simulink model "Final_Microgrid_Ssstem"  (R2021a)
settings: Solver=VariableStepAuto  StartTime=0.0  StopTime=.2  RelTol=1e-3
undefined symbols (not defined in the file): Acid, Lead
libraries: spsIGBTDiodeLib x6, spsSeriesRLCBranchLib x3, spsVoltageMeasurementLib x3, spsCurrentMeasurementLib x2, spsACVoltageSourceLib x1, spsBatteryLib x1, pid_lib x1, spsPLLLib x1, spsPWMGeneratorDCDCLib x1, spspowerguiLib x1
settings Model: Creator=User  LastModifiedBy=User
settings SolverCC: AlgebraicLoopSolver=TrustRegion
settings DataIOCC: ReturnWorkspaceOutputs=off
settings DebuggingCC: SFMachineParentedDataDiag=warning  ArithmeticOperatorsInVariantConditions=warning
settings SFSimCC: SimUseLocalCustomCode=off  CustomCodeUndefinedFunction=UseInterfaceOnly
settings RTWCC: RTWUseLocalCustomCode=off

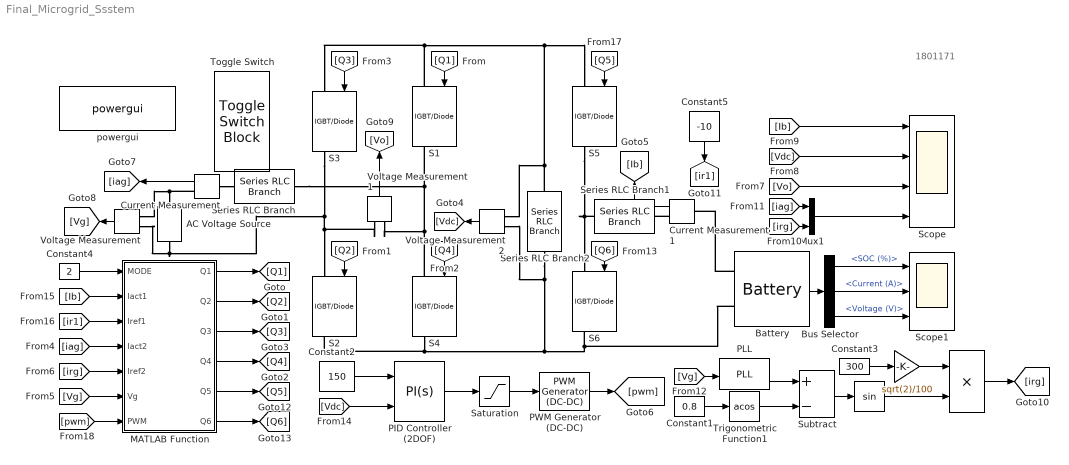
== system Final_Microgrid_Ssstem ==
  note: 1801171
  " " : Product
  "  " : Gain  Gain=sqrt(2)/100
  "   " : Trigonometry
  AC Voltage Source : spsACVoltageSourceLib/AC Voltage Source  Amplitude=100*sqrt(2)  Phase=0  Frequency=50  SampleTime=0  Measurements=None  BusType=swing  Pref=10e3  Qref=0  Qmin=-inf  Qmax=+inf
  Battery : spsBatteryLib/Battery  BatType=Lead-Acid  ShowTempParam=off  ThermalPreset=no  ShowAgeParam=off  NomV=60  NomQ=5.4  SOC=100  Batt_Tr=30  PresetModel=off  MaxQ=5.4  MinV=45  FullV=80  Dis_rate=2.3478  R=0.013333  Normal_OP=4.8835  expZone="[70      0.2653]"  current=[6.5 13 32.5]  Units=Time  Tci=20  NomT=20  T2=-30  MaxQ2=4.8  FullV2=7.1  Normal_OP2=5.655  expZone2="[6.58           1]"  Rca=0.6  ti=2000  Dp=0  Neq0=0  Tsim=1e6  Ta1=25  Qeol=5.4*0.9  Reol=0.013333*1.2  Char_age=[2.3478, 3]  Dis_age=[2.3478, 10]  N1=1500  N2=10500  N3=1000  N4=1400  Ta2=45  N5=950
  Bus Selector : BusSelector  OutputSignals=SOC (%),Current (A),Voltage (V)
  Constant1 : Constant  Value=0.8
  Constant2 : Constant  Value=150
  Constant3 : Constant  Value=300
  Constant4 : Constant  Value=2
  Constant5 : Constant  Value=-10
  Current Measurement : spsCurrentMeasurementLib/Current Measurement  PhasorSimulation=off  OutputType=Complex  PSBequivalent=0
  Current Measurement1 : spsCurrentMeasurementLib/Current Measurement  PhasorSimulation=off  OutputType=Complex  PSBequivalent=0
  MATLAB Function : MATLAB Function  TreatAsAtomicUnit=on
  Mux1 : Mux  Inputs=2
  PID Controller (2DOF) : pid_lib/PID Controller (2DOF)  Controller=PI  Form=Parallel  TimeDomain=Continuous-time  UseExternalTs=off  SampleTime=-1  IntegratorMethod=Forward Euler  FilterMethod=Forward Euler  ControllerParametersSource=internal  P=0.1  I=0.01  D=0  UseFilter=on  N=100  b=1  c=1  TunerSelectOption=Transfer Function Based (PID Tuner App)  InitialConditionSource=internal  InitialConditionForIntegrator=0  InitialConditionForFilter=0  DifferentiatorICPrevScaledInput=0  ExternalReset=none  TrackingMode=off  Kt=1  LimitOutput=off  SatLimitsSource=internal  UpperSaturationLimit=inf  LowerSaturationLimit=-inf  LinearizeAsGain=on  AntiWindupMode=none  Kb=1  POutMin=[]  POutMax=[]  IOutMin=[]  IOutMax=[]  DOutMin=[]  DOutMax=[]  NOutMin=[]  NOutMax=[]  bOutMin=[]  bOutMax=[]  cOutMin=[]  cOutMax=[]  SumOutMin=[]  SumOutMax=[]  SaturationOutMin=[]  SaturationOutMax=[]  PParamMin=[]  PParamMax=[]  IParamMin=[]  IParamMax=[]  DParamMin=[]  DParamMax=[]  NParamMin=[]  NParamMax=[]  bParamMin=[]  bParamMax=[]  cParamMin=[]  cParamMax=[]  KbParamMin=[]  KbParamMax=[]  KtParamMin=[]  KtParamMax=[]  KbOutMin=[]  KbOutMax=[]  KtOutMin=[]  KtOutMax=[]  IntegratorOutMin=[]  IntegratorOutMax=[]  FilterOutMin=[]  FilterOutMax=[]  SumI1OutMin=[]  SumI1OutMax=[]  SumI2OutMin=[]  SumI2OutMax=[]  SumI3OutMin=[]  SumI3OutMax=[]  SumI4OutMin=[]  SumI4OutMax=[]  SumDOutMin=[]  SumDOutMax=[]  Sum1OutMin=[]  Sum1OutMax=[]  Sum2OutMin=[]  Sum2OutMax=[]  Sum3OutMin=[]  Sum3OutMax=[]  DifferentiatorOutMin=[]  DifferentiatorOutMax=[]  FilterDiffOutCoefMin=[]  FilterDiffOutCoefMax=[]  ReciprocalOutMin=[]  ReciprocalOutMax=[]  SumDenOutMin=[]  SumDenOutMax=[]  SumNumOutMin=[]  SumNumOutMax=[]  DivideOutMin=[]  DivideOutMax=[]  UdiffTsProdOutMin=[]  UdiffTsProdOutMax=[]  NTsProdOutMin=[]  NTsProdOutMax=[]  UintegralTsProdOutMin=[]  UintegralTsProdOutMax=[]  UngainTsProdOutMin=[]  UngainTsProdOutMax=[]  IntegratorContinuousStateAttributes=''  IntegratorStateMustResolveToSignalObject=off  IntegratorRTWStateStorageClass=Auto  FilterContinuousStateAttributes=''  FilterStateMustResolveToSignalObject=off  FilterRTWStateStorageClass=Auto  ParallelPVariant=InternalParameters  IdealPVariant=Disabled  IVariant=InternalParameters  DVariant=Disabled  bVariant=InternalParameters  cVariant=Disabled  IntegratorVariant=Continuous  SatVariant=Disabled  AWVariant=Passthrough  PCopyVariant=Disabled  TRVariant=Disabled  FdbkBlocksVariant=Forward  IdealPFdbkVariant=Disabled  SatFdbkVariant=Disabled  DerivativeFilterVariant=Disabled  NVariant=Disabled  NCopyVariant=Disabled_SignalSpec  FilterICVariant=Disabled  IntegratorICVariant=InternalICs  ExternalResetVariant=Disabled  TRSumVariant=Passthrough  SumFdbkVariant=Disabled  SumVariant=Sum_PI  TsampFilterVariant=InternalTs  TsampNgainVariant=Passthrough  TsampIntegralVariant=Passthrough  ExternalSaturationOutDataTypeStr=Inherit: Same as second input
      settings: SourceProductBaseCode=SL
  PLL : spsPLLLib/PLL  Fmin=45  Par_Init=[0, 50]  ParK=[180, 3200, 1]  TcD=1e-4  MaxRateChangeFreq=12  FilterCutOffFreq=25  Ts=0  AGC=on
      settings: SourceProductBaseCode=PS
  PWM Generator (DC-DC) : spsPWMGeneratorDCDCLib/PWM Generator (DC-DC)  Fsw=5000  Ts=0
  S{1..6} (6 alike) : spsIGBTDiodeLib/IGBT//Diode  Ron=1e-3  Rs=1e5  Cs=inf  Measurements=on
  Saturation : Saturate  LowerLimit=0
  Scope : Scope  NumInputPorts=4
  Scope1 : Scope  NumInputPorts=3
  Series RLC Branch : spsSeriesRLCBranchLib/Series RLC Branch  LConnTagsString=__new0  RConnTagsString=__new0  BranchType=RL  Resistance=.1  Inductance=5e-3  SetiL0=off  InitialCurrent=0  Capacitance=1e-6  Setx0=off  InitialVoltage=0  Measurements=Branch voltage and current
  Series RLC Branch1 : spsSeriesRLCBranchLib/Series RLC Branch  LConnTagsString=__new0  RConnTagsString=__new0  BranchType=RL  Resistance=.1  Inductance=5e-3  SetiL0=off  InitialCurrent=0  Capacitance=1e-6  Setx0=off  InitialVoltage=0  Measurements=Branch voltage and current
  Series RLC Branch2 : spsSeriesRLCBranchLib/Series RLC Branch  LConnTagsString=__new0  RConnTagsString=__new0  BranchType=C  Resistance=.1  Inductance=5e-3  SetiL0=off  InitialCurrent=0  Capacitance=1000e-6  Setx0=off  InitialVoltage=0  Measurements=Branch voltage and current
  Subtract : Sum  Inputs=+-
  Toggle Switch : ToggleSwitchBlock
      settings: Values={{'Off', 'On'}, [1 2]}
  Trigonometric Function1 : Trigonometry  Operator=acos
  Voltage Measurement : spsVoltageMeasurementLib/Voltage Measurement  PhasorSimulation=off  OutputType=Complex  PSBequivalent=0
  Voltage Measurement1 : spsVoltageMeasurementLib/Voltage Measurement  PhasorSimulation=off  OutputType=Complex  PSBequivalent=0
  Voltage Measurement2 : spsVoltageMeasurementLib/Voltage Measurement  PhasorSimulation=off  OutputType=Complex  PSBequivalent=0
  powergui : spspowerguiLib/powergui  Priority=1  SimulationMode=Discrete  SampleTime=0.5e-6  frequency=60  Iterations=50  frequencyindice=0  Pbase=100e6  ErrMax=1e-4  UnitsV=kV  UnitsW=MW  buscounter=0  FunctionMessages=off  echomessages=off  EnableUseOfTLC=off  CurrentSourceSwitches=off  DisableSnubberDevices=off  DisableRonSwitches=off  DisableVfSwitches=off  DisplayEquations=off  AutomaticDiscreteSolvers=off  SolverType=Tustin/Backward Euler (TBE)  Interpol=off  ExternalGateDelay=off  methode=off  Ts=100  x0status=blocks  SPID=on  SwTol=0  HookPort=off  NonlinearTolerance=1e-4  nMaxIteration=100  ContinueOnMaxIteration=off  RestoreLinks=warning  ResistiveCurrentMeasurement=off  Frange=[0:2:500]  Ylog=off  Xlog=on  ShowGrid=off  save=off  variable=ZData  structure=0  ZoomFFT=off  StartTime=0.0  cycles=1  DisplayStyle=1  fundamental=60  FreqAxis=off  MaxFrequency=1000  frequencyindicesteady=1  RmsSteady=1  display=off
  wires:
  MATLAB Function/1(Q1) -> [Q1]
  MATLAB Function/2(Q2) -> [Q2]
  MATLAB Function/3(Q3) -> [Q3]
  MATLAB Function/4(Q4) -> [Q4]
  [Q1] -> S1/1
  [Q2] -> S2/1
  [Q4] -> S4/1
  [Q3] -> S3/1
  [Vg] -> MATLAB Function/6(Vg)
  Current Measurement/1 -> [iag]
  Voltage Measurement/1 -> [Vg]
  Voltage Measurement1/1 -> [Vo]
  [Vg] -> PLL/1
  Constant1/1 -> Trigonometric Function1/1
  Trigonometric Function1/1 -> Subtract/2
  PLL/2 -> Subtract/1
  Subtract/1 -> "   "/1
  Constant3/1 -> "  "/1
  Mux1/1 -> Scope/4
  [iag] -> Mux1/1
  [irg] -> Mux1/2
  " "/1 -> [irg]
  "  "/1 -> " "/1
  "   "/1 -> " "/2
  Constant2/1 -> PID Controller (2DOF)/1
  Voltage Measurement2/1 -> [Vdc]
  [Vo] -> Scope/3
  [Vdc] -> Scope/2
  Current Measurement1/1 -> [Ib]
  [Ib] -> Scope/1
  PWM Generator (DC-DC)/1 -> [pwm]
  [Vdc] -> PID Controller (2DOF)/2
  PID Controller (2DOF)/1 -> Saturation/1
  Saturation/1 -> PWM Generator (DC-DC)/1
  Constant4/1 -> MATLAB Function/1(MODE)
  Constant5/1 -> [ir1]
  MATLAB Function/5(Q5) -> [Q5]
  MATLAB Function/6(Q6) -> [Q6]
  [Q5] -> S5/1
  [pwm] -> MATLAB Function/7(PWM)
  [Q6] -> S6/1
  [iag] -> MATLAB Function/4(Iact2)
  [irg] -> MATLAB Function/5(Iref2)
  [Ib] -> MATLAB Function/2(Iact1)
  [ir1] -> MATLAB Function/3(Iref1)
  Battery/1 -> Bus Selector/1
  Bus Selector/2 -> Scope1/2  "<Current (A)>"
  Bus Selector/1 -> Scope1/1  "<SOC (%)>"
  Bus Selector/3 -> Scope1/3  "<Voltage (V)>"
  connections:
  S3/RConn1 -- Voltage Measurement1/LConn2 -- S2/LConn1 -- AC Voltage Source/LConn1 -- Voltage Measurement/LConn2
  Current Measurement/LConn1 -- Series RLC Branch/RConn1
  S4/LConn1 -- Voltage Measurement1/LConn1 -- Series RLC Branch/LConn1 -- S1/RConn1
  Current Measurement/RConn1 -- Voltage Measurement/LConn1 -- AC Voltage Source/RConn1
  S5/RConn1 -- S6/LConn1 -- Series RLC Branch1/RConn1
  S4/RConn1 -- Series RLC Branch2/RConn1 -- Voltage Measurement2/LConn2 -- Battery/LConn2 -- S6/RConn1 -- S2/RConn1
  Battery/LConn1 -- Current Measurement1/LConn1
  Current Measurement1/RConn1 -- Series RLC Branch1/LConn1
  S1/LConn1 -- Series RLC Branch2/LConn1 -- Voltage Measurement2/LConn1 -- S5/LConn1 -- S3/LConn1

== matlab function Final_Microgrid_Ssstem/MATLAB Function ==
  settings: updateMethod=DISCRETE
  data: MODE input; Iact1 input; Q1 output; Iref1 input; Iact2 input; Iref2 input; Q2 output; Q3 output; Q4 output; Vg input; Q5 output; Q6 output; PWM input
function [Q1,Q2,Q3,Q4,Q5,Q6] = fcn(MODE,Iact1,Iref1,Iact2,Iref2,Vg,PWM)
persistent S1
if isempty(S1);S1=0;end
persistent S2
if isempty(S2);S2=0;end
persistent S3
if isempty(S3);S3=0;end
persistent S4
if isempty(S4);S4=0;end
persistent S5
if isempty(S5);S5=1;end
persistent S6
if isempty(S6);S6=0;end
if MODE==1
    S1=0;S2=0;S3=0;S4=0;S6=0;
    e1=Iact1-Iref1;
    d1=0.5;
    if e1>=d1
        S5=1;
    elseif e1<=-d1
        S5=0;
    else S5=S5;
    end
 
else MODE==2
    d2=0.5;
    S6=PWM;
    S5=0;
    e2=Iact2-Iref2;
    if Vg>=0
        if e2<=-d2
            S1=1;S2=1;S3=0;S4=0;
        elseif e2>=d2
            S1=1;S2=0;S3=1;S4=0;
        else
            S1 = S1;S2=S2;S3=S3;S4=S4;
        end
    else
        if e2<=-d2
            S1=0;S2=1;S3=0;S4=1;
        elseif e2>=d2
            S1=0;S2=0;S3=1;S4=1;
        else
            S1 = S1;S2=S2;S3=S3;S4=S4;
        end
    end
end
Q1=S1; Q2=S2; Q3=S3; Q4=S4;Q5=S5;Q6=S6;
end
